simulink model "FM&PM_Simulink"  (R2021a)
settings: Solver=VariableStepAuto  StartTime=0.0  StopTime=2  RelTol=1e-3
libraries: commanabbnd3 x4
settings Model: Creator=DAN  LastModifiedBy=DAN

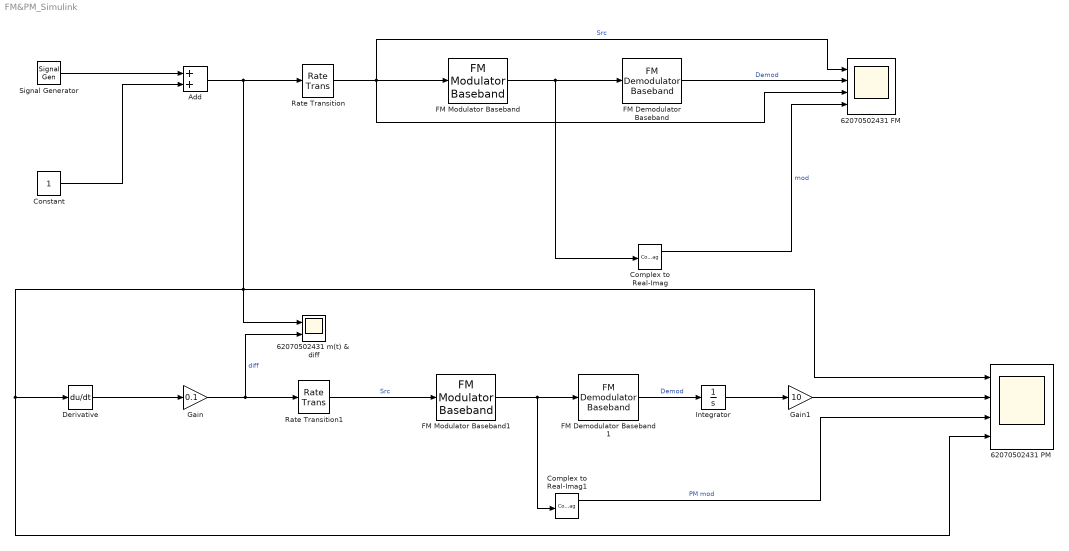
== system FM&PM_Simulink ==
  62070502431 FM : Scope  NumInputPorts=4
  62070502431 PM : Scope  NumInputPorts=4
  62070502431 m(t) & diff : Scope  NumInputPorts=2
  Add : Sum
  Complex to Real-Imag : ComplexToRealImag
  Complex to Real-Imag1 : ComplexToRealImag
  Constant : Constant
  Derivative : Derivative
  "FM Demodulator Baseband " : commanabbnd3/FM Demodulator Baseband   FrequencyDeviation=50  SimulateUsing=Code generation
      settings: SourceProductBaseCode=CM
  FM Demodulator Baseband 1 : commanabbnd3/FM Demodulator Baseband   FrequencyDeviation=50  SimulateUsing=Code generation
      settings: SourceProductBaseCode=CM
  FM Modulator Baseband : commanabbnd3/FM Modulator Baseband  FrequencyDeviation=50  SimulateUsing=Code generation
      settings: SourceProductBaseCode=CM
  FM Modulator Baseband1 : commanabbnd3/FM Modulator Baseband  FrequencyDeviation=50  SimulateUsing=Code generation
      settings: SourceProductBaseCode=CM
  Gain : Gain  Gain=0.1
  Gain1 : Gain  Gain=10
  Integrator : Integrator
  Rate Transition : RateTransition  OutPortSampleTime=0.000001
  Rate Transition1 : RateTransition  OutPortSampleTime=0.000001
  Signal Generator : SignalGenerator  WaveForm=sawtooth  Frequency=4
  wires:
  Signal Generator/1 -> Add/1
  Constant/1 -> Add/2
  Add/1 -> Rate Transition/1, 62070502431 PM/4, Derivative/1, 62070502431 PM/1, 62070502431 m(t) & diff/1
  Rate Transition/1 -> 62070502431 FM/3, 62070502431 FM/1, FM Modulator Baseband/1  "Src"
  FM Modulator Baseband/1 -> Complex to Real-Imag/1, "FM Demodulator Baseband "/1
  "FM Demodulator Baseband "/1 -> 62070502431 FM/2  "Demod"
  Complex to Real-Imag/1 -> 62070502431 FM/4  "mod"
  Gain/1 -> 62070502431 m(t) & diff/2, Rate Transition1/1  "diff"
  Rate Transition1/1 -> FM Modulator Baseband1/1  "Src"
  FM Modulator Baseband1/1 -> Complex to Real-Imag1/1, FM Demodulator Baseband 1/1
  FM Demodulator Baseband 1/1 -> Integrator/1  "Demod"
  Integrator/1 -> Gain1/1
  Gain1/1 -> 62070502431 PM/2
  Derivative/1 -> Gain/1
  Complex to Real-Imag1/1 -> 62070502431 PM/3  "PM mod"
